simulink library "windowed_limit_lib"  (R2012b)
settings: Solver=ode45  StartTime=0.0  StopTime=10.0  RelTol=1e-3
settings Model: Creator=CH24070  LastModifiedBy=CH24070

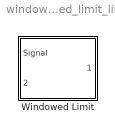
== system windowed_limit_lib ==
  Windowed Limit : Subsystem

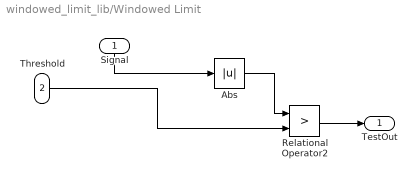
== system windowed_limit_lib/Windowed Limit ==
  Signal : Inport
  Threshold : Inport  Port=2
  Abs : Abs
  Relational Operator2 : RelationalOperator  Operator=>  OutDataTypeStr=boolean
  TestOut : Outport
  wires:
  Abs/1 -> Relational Operator2/1
  Relational Operator2/1 -> TestOut/1
  Threshold/1 -> Relational Operator2/2
  Signal/1 -> Abs/1
